simulink model "simpleVehicleModel_Trial2"  (R2017b)
settings: Solver=FixedStepAuto  StartTime=0.0  StopTime=inf  FixedStep=0.01  RelTol=1e-3
values from neighbouring files (symbols this model uses):
  beta_ref = 20*pi/180    (= 0.349065850399)    [initialize_simplemodel_Trial.m]
  g = 9.81    [initialize_simplemodel.m]    (also in initialize_simplemodel_Trial.m; tire_friction_circle.m)
  h = 0.35    [initialize_simplemodel.m]    (also in initialize_simplemodel_Trial.m)
  Izz = 1800    [initialize_simplemodel.m]    (also in initialize_simplemodel_Trial.m = 1400)
  lf = 1.4    [initialize_simplemodel.m]    (also in initialize_simplemodel_Trial.m)
  lr = 1.345    [initialize_simplemodel.m]    (also in initialize_simplemodel_Trial.m)
  m = 1400    [initialize_simplemodel.m]    (also in initialize_simplemodel_Trial.m = 1300; tire_friction_circle.m = 1300)
  r = 0.34    [initialize_simplemodel.m]    (also in initialize_simplemodel_Trial.m)
  tr = 1.684/2    (= 0.842)    [initialize_simplemodel.m]    (also in initialize_simplemodel_Trial.m)
  vx = 10    [initialize_simplemodel_Trial.m]    (also in pp_from_simple_model.m; tire_friction_circle.m = 5)
undefined symbols (not defined in the file or in its folder): DiscIntNeverNeededParam
libraries: simulink x35
(part 1 of 2)
settings Model: Creator=ashwin.ramanujam  LastModifiedBy=gandh

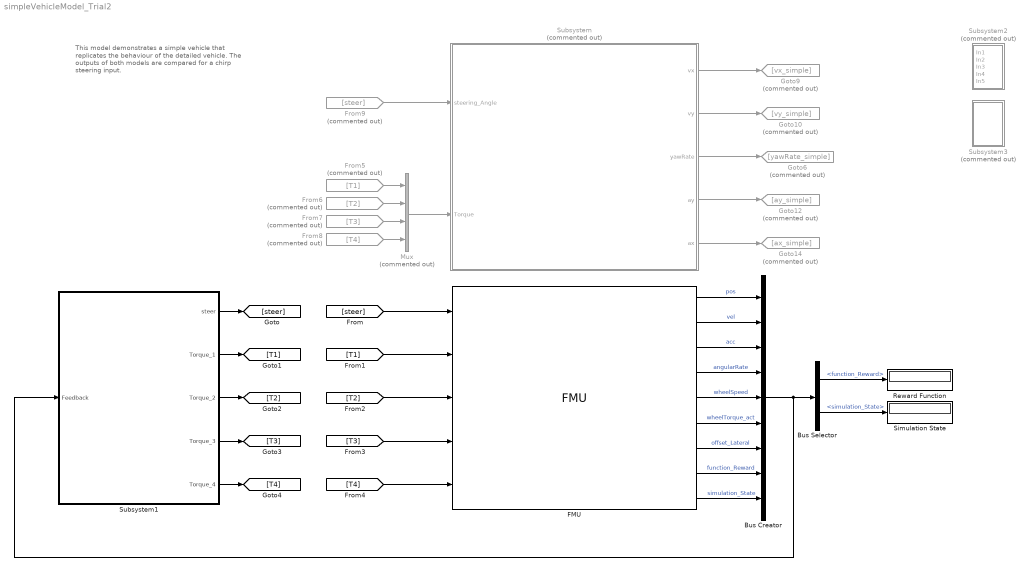
== system simpleVehicleModel_Trial2 ==
  note: This model demonstrates a simple vehicle that replicates the behaviour of the detailed vehicle. The outputs of both models are compared for a chirp steering input.
  Bus Creator : BusCreator  Inputs=9
  Bus Selector : BusSelector  OutputSignals=function_Reward,simulation_State
  FMU : FMU  FMUName=MED2018_VehicleModel.fmu  FMUMode=CoSimulation  FMUSampleTime=-1  mask(MED2018.VehicleModel [Co-Simulation, v2.0]){}
  From5 : From  Commented=on  GotoTag=T1
  From6 : From  Commented=on  GotoTag=T2
  From7 : From  Commented=on  GotoTag=T3
  From8 : From  Commented=on  GotoTag=T4
  From9 : From  Commented=on  GotoTag=steer
  Goto10 : Goto  Commented=on  GotoTag=vy_simple
  Goto12 : Goto  Commented=on  GotoTag=ay_simple
  Goto14 : Goto  Commented=on  GotoTag=ax_simple
  Goto6 : Goto  Commented=on  GotoTag=yawRate_simple
  Goto9 : Goto  Commented=on  GotoTag=vx_simple
  Mux : Mux  Commented=on
  Reward Function : Display
  Simulation State : Display
  Subsystem : Subsystem  Commented=on
  Subsystem1 : Subsystem
  Subsystem2 : Subsystem  Commented=on
  Subsystem3 : Subsystem  Commented=on
  wires:
  Mux/1 -> Subsystem/2(Torque)
  [steer] -> FMU/1
  [T4] -> FMU/5
  [T1] -> FMU/2
  [T2] -> FMU/3
  [T3] -> FMU/4
  From5/1 -> Mux/1
  From6/1 -> Mux/2
  From7/1 -> Mux/3
  From8/1 -> Mux/4
  Subsystem/3(yawRate) -> Goto6/1
  Subsystem/1(vx) -> Goto9/1
  Subsystem/2(vy) -> Goto10/1
  Subsystem/4(ay) -> Goto12/1
  Subsystem/5(ax) -> Goto14/1
  From9/1 -> Subsystem/1(steering_Angle)
  Subsystem1/1(steer) -> [steer]
  Subsystem1/2(Torque_1) -> [T1]
  Subsystem1/3(Torque_2) -> [T2]
  Subsystem1/4(Torque_3) -> [T3]
  Subsystem1/5(Torque_4) -> [T4]
  FMU/1 -> Bus Creator/1  "pos"
  FMU/6 -> Bus Creator/6  "wheelTorque_act"
  FMU/8 -> Bus Creator/8  "function_Reward"
  FMU/3 -> Bus Creator/3  "acc"
  FMU/5 -> Bus Creator/5  "wheelSpeed"
  FMU/7 -> Bus Creator/7  "offset_Lateral"
  FMU/2 -> Bus Creator/2  "vel"
  FMU/4 -> Bus Creator/4  "angularRate"
  FMU/9 -> Bus Creator/9  "simulation_State"
  Bus Creator/1 -> Subsystem1/1(Feedback), Bus Selector/1
  Bus Selector/1 -> Reward Function/1  "<function_Reward>"
  Bus Selector/2 -> Simulation State/1  "<simulation_State>"

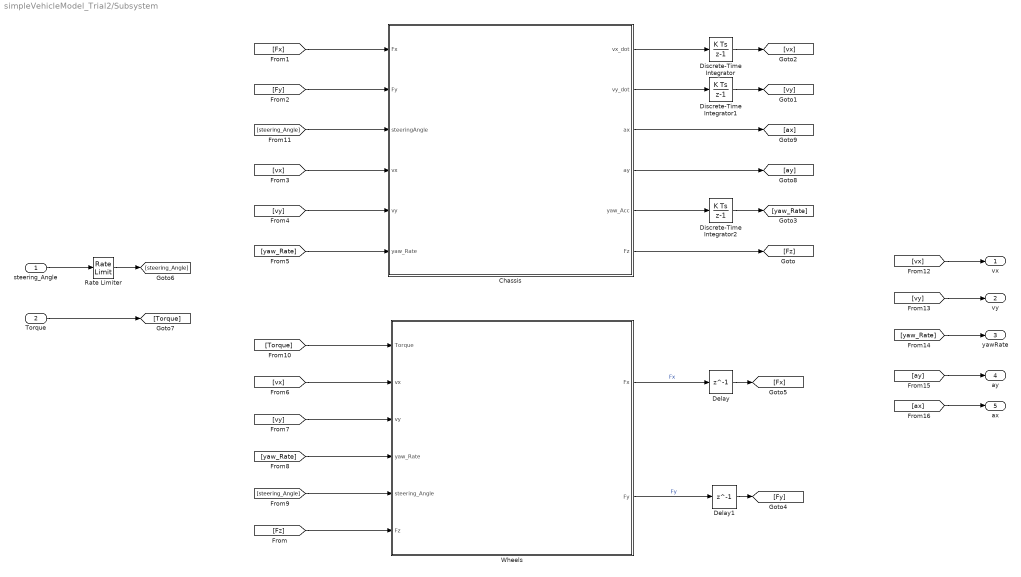
== system simpleVehicleModel_Trial2/Subsystem ==
  steering_Angle : Inport
  Torque : Inport  Port=2
  Chassis : MATLAB Function  TreatAsAtomicUnit=on
  Delay : Delay  DelayLength=1  InitialCondition=[m*g*lr/(lf+lr)/2;m*g*lr/(lf+lr)/2;m*g*lf/(lf+lr)/2;m*g*lf/(lf+lr)/2]
  Delay1 : Delay  DelayLength=1  InitialCondition=[m*g*lr/(lf+lr)/2;m*g*lr/(lf+lr)/2;m*g*lf/(lf+lr)/2;m*g*lf/(lf+lr)/2]
  Discrete-Time Integrator : DiscreteIntegrator  InitialCondition=60*5/18  InitialConditionSetting=State (most efficient)  SampleTime=-1  ICPrevOutput=DiscIntNeverNeededParam  ICPrevScaledInput=DiscIntNeverNeededParam
  Discrete-Time Integrator1 : DiscreteIntegrator  InitialConditionSetting=State (most efficient)  SampleTime=-1  ICPrevOutput=DiscIntNeverNeededParam  ICPrevScaledInput=DiscIntNeverNeededParam
  Discrete-Time Integrator2 : DiscreteIntegrator  InitialConditionSetting=State (most efficient)  SampleTime=-1  ICPrevOutput=DiscIntNeverNeededParam  ICPrevScaledInput=DiscIntNeverNeededParam
  Rate Limiter : RateLimiter  RisingSlewLimit=500*pi/180/12  FallingSlewLimit=-500*pi/180/12  SampleTimeMode=inherited
  Wheels : Subsystem  Priority=0
  vx : Outport
  vy : Outport  Port=2
  yawRate : Outport  Port=3
  ay : Outport  Port=4
  ax : Outport  Port=5
  wires:
  [vx] -> Chassis/4(vx)
  Discrete-Time Integrator2/1 -> [yaw_Rate]
  [Fy] -> Chassis/2(Fy)
  [vy] -> Wheels/3(vy)
  [Torque] -> Wheels/1(Torque)
  [yaw_Rate] -> yawRate/1
  [yaw_Rate] -> Wheels/4(yaw_Rate)
  [vx] -> vx/1
  [vx] -> Wheels/2(vx)
  [Fz] -> Wheels/6(Fz)
  [steering_Angle] -> Chassis/3(steeringAngle)
  [steering_Angle] -> Wheels/5(steering_Angle)
  steering_Angle/1 -> Rate Limiter/1
  Torque/1 -> [Torque]
  [vy] -> vy/1
  Chassis/5(yaw_Acc) -> Discrete-Time Integrator2/1
  Wheels/1(Fx) -> Delay/1  "Fx"
  Wheels/2(Fy) -> Delay1/1  "Fy"
  Chassis/6(Fz) -> [Fz]
  [ay] -> ay/1
  Delay/1 -> [Fx]
  Delay1/1 -> [Fy]
  Chassis/1(vx_dot) -> Discrete-Time Integrator/1
  Chassis/4(ay) -> [ay]
  Chassis/3(ax) -> [ax]
  [ax] -> ax/1
  Chassis/2(vy_dot) -> Discrete-Time Integrator1/1
  [vy] -> Chassis/5(vy)
  [yaw_Rate] -> Chassis/6(yaw_Rate)
  [Fx] -> Chassis/1(Fx)
  Discrete-Time Integrator1/1 -> [vy]
  Discrete-Time Integrator/1 -> [vx]
  Rate Limiter/1 -> [steering_Angle]

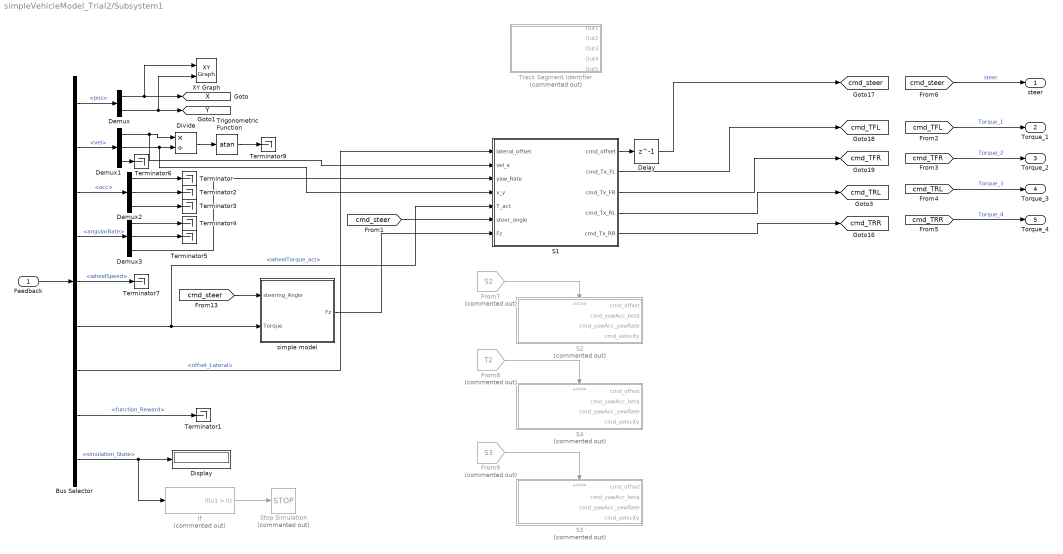
== system simpleVehicleModel_Trial2/Subsystem1 ==
  Feedback : Inport
  Bus Selector : BusSelector  OutputSignals=pos,vel,acc,angularRate,wheelSpeed,wheelTorque_act,offset_Lateral,function_Reward,simulation_State
  Delay : Delay  DelayLength=1
  Demux : Demux  Outputs=2
  Demux1 : Demux  Outputs=3
  Demux2 : Demux  Outputs=3
  Demux3 : Demux  Outputs=3
  Display : Display
  Divide : Product  Inputs=*/
  From7 : From  Commented=on  GotoTag=S2  TagVisibility=global
  From8 : From  Commented=on  GotoTag=T2  TagVisibility=global
  From9 : From  Commented=on  GotoTag=S3  TagVisibility=global
  If : If  Commented=on  ShowElse=off
  S1 : Subsystem  TreatAsAtomicUnit=on
  S2 : Subsystem  Commented=on  TreatAsAtomicUnit=on
  S3 : Subsystem  Commented=on  TreatAsAtomicUnit=on
  S4 : Subsystem  Commented=on  TreatAsAtomicUnit=on
  Stop Simulation : Stop  Commented=on
  Terminator{,1..7,9} (9 alike) : Terminator
  Track Segment Identifier : Subsystem  Commented=on
  Trigonometric Function : Trigonometry  Operator=atan
  XY Graph : simulink/Sinks/XY Graph  xmin=-5  xmax=110  ymin=-10  ymax=180  st=-1
  simple model : Subsystem
  steer : Outport
  Torque_1 : Outport  Port=2
  Torque_2 : Outport  Port=3
  Torque_3 : Outport  Port=4
  Torque_4 : Outport  Port=5
  tag scope: X=global, Y=global, cmd_TFL=global, cmd_TFR=global, cmd_TRL=global, cmd_TRR=global, cmd_steer=global
  wires:
  [cmd_TFL] -> Torque_1/1  "Torque_1"
  [cmd_TRL] -> Torque_3/1  "Torque_3"
  [cmd_TFR] -> Torque_2/1  "Torque_2"
  [cmd_TRR] -> Torque_4/1  "Torque_4"
  [cmd_steer] -> steer/1  "steer"
  Feedback/1 -> Bus Selector/1
  Bus Selector/1 -> Demux/1  "<pos>"
  Demux/2 -> XY Graph/2, [Y]
  Demux/1 -> XY Graph/1, [X]
  Demux1/1 -> S1/2(vel_x), Divide/1
  Bus Selector/2 -> Demux1/1  "<vel>"
  Demux2/3 -> Terminator3/1
  Bus Selector/3 -> Demux2/1  "<acc>"
  Demux2/2 -> Terminator2/1
  Demux2/1 -> Terminator/1
  Demux3/1 -> Terminator4/1
  Demux3/2 -> Terminator5/1
  Bus Selector/4 -> Demux3/1  "<angularRate>"
  Demux3/3 -> S1/3(yaw_Rate)
  Bus Selector/5 -> Terminator7/1  "<wheelSpeed>"
  Bus Selector/8 -> Terminator1/1  "<function_Reward>"
  Bus Selector/9 -> If/1, Display/1  "<simulation_State>"
  Demux1/2 -> S1/4(v_y), Divide/2
  Divide/1 -> Trigonometric Function/1
  Trigonometric Function/1 -> Terminator9/1
  If/1 -> Stop Simulation/1
  From7/1 -> S2/Action
  From8/1 -> S4/Action
  From9/1 -> S3/Action
  Demux1/3 -> Terminator6/1
  Bus Selector/6 -> S1/5(T_act), simple model/2(Torque)  "<wheelTorque_act>"
  [cmd_steer] -> simple model/1(steering_Angle)
  [cmd_steer] -> S1/6(steer_angle)
  simple model/1(Fz) -> S1/7(Fz)
  Bus Selector/7 -> S1/1(lateral_offset)  "<offset_Lateral>"
  S1/2(cmd_Tx_FL) -> [cmd_TFL]
  S1/3(cmd_Tx_FR) -> [cmd_TFR]
  S1/4(cmd_Tx_RL) -> [cmd_TRL]
  S1/5(cmd_Tx_RR) -> [cmd_TRR]
  S1/1(cmd_offset) -> Delay/1
  Delay/1 -> [cmd_steer]

== system simpleVehicleModel_Trial2/Subsystem2 ==
  In1 : Inport
  In2 : Inport  Port=2
  In3 : Inport  Port=3
  In4 : Inport  Port=4
  In5 : Inport  Port=5
  Demux : Demux  Commented=on  Outputs=3
  Demux1 : Demux  Commented=on  Outputs=3
  Demux2 : Demux  Commented=on  Outputs=3
  Demux3 : Demux  Commented=on  Outputs=2
  Goto11 : Goto  Commented=on  GotoTag=ay_FMU
  Goto13 : Goto  Commented=on  GotoTag=ax_FMU
  Goto15 : Goto  Commented=on  GotoTag=offset_Lateral  TagVisibility=global
  Goto5 : Goto  Commented=on  GotoTag=yawRate_FMU
  Goto7 : Goto  Commented=on  GotoTag=vx_FMU
  Goto8 : Goto  Commented=on  GotoTag=vy_FMU
  Terminator{,2..4} (4 alike) : Terminator  Commented=on
  XY Graph : simulink/Sinks/XY Graph  Commented=on  xmin=-5  xmax=110  ymin=-10  ymax=180  st=-1
  wires:
  Demux/3 -> Goto5/1
  Demux1/1 -> Goto7/1
  Demux1/2 -> Goto8/1
  Demux/1 -> Terminator3/1
  Demux/2 -> Terminator4/1
  Demux2/2 -> Goto11/1
  Demux1/3 -> Terminator/1
  Demux2/1 -> Goto13/1
  Demux3/1 -> XY Graph/1
  Demux3/2 -> XY Graph/2
  Demux2/3 -> Terminator2/1
  In5/1 -> Goto15/1
  In2/1 -> Demux1/1
  In4/1 -> Demux/1
  In1/1 -> Demux3/1
  In3/1 -> Demux2/1

== system simpleVehicleModel_Trial2/Subsystem3 ==
  Scope{,1..3,5} (5 alike) : Scope  NumInputPorts=2
  wires:
  [vx_simple] -> Scope/1  "vx_simple"
  [vx_FMU] -> Scope/2  "vx_FMU"
  [vy_FMU] -> Scope1/2  "vy_FMU"
  [vy_simple] -> Scope1/1  "vy_simple"
  [ax_FMU] -> Scope5/2  "ax_FMU"
  [yawRate_simple] -> Scope2/1  "yawRate_simple"
  [yawRate_FMU] -> Scope2/2  "yawRate_FMU"
  [ay_simple] -> Scope3/1  "ay_simple"
  [ay_FMU] -> Scope3/2  "ay_FMU"
  [ax_simple] -> Scope5/1  "ax_simple"

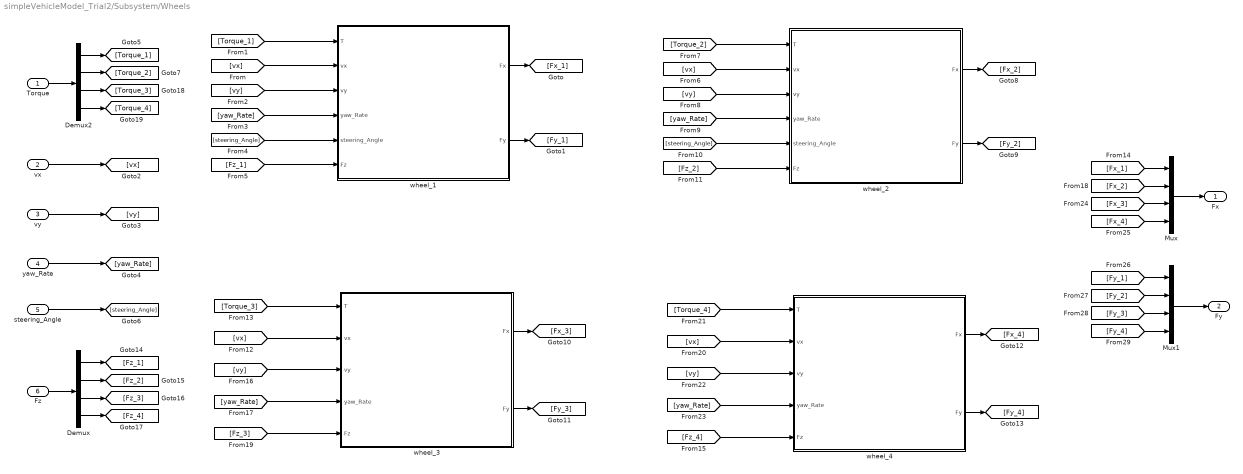
== system simpleVehicleModel_Trial2/Subsystem/Wheels ==
  Torque : Inport
  vx : Inport  Port=2
  vy : Inport  Port=3
  yaw_Rate : Inport  Port=4
  steering_Angle : Inport  Port=5
  Fz : Inport  Port=6
  Demux : Demux
  Demux2 : Demux
  Mux : Mux
  Mux1 : Mux
  wheel_1 : Subsystem
  wheel_2 : Subsystem
  wheel_3 : Subsystem
  wheel_4 : Subsystem
  Fx : Outport
  Fy : Outport  Port=2
  wires:
  vx/1 -> [vx]
  vy/1 -> [vy]
  yaw_Rate/1 -> [yaw_Rate]
  [vx] -> wheel_1/2(vx)
  wheel_1/1(Fx) -> [Fx_1]
  wheel_1/2(Fy) -> [Fy_1]
  [steering_Angle] -> wheel_1/5(steering_Angle)
  [yaw_Rate] -> wheel_1/4(yaw_Rate)
  [vy] -> wheel_1/3(vy)
  [Torque_1] -> wheel_1/1(T)
  steering_Angle/1 -> [steering_Angle]
  wheel_2/1(Fx) -> [Fx_2]
  wheel_2/2(Fy) -> [Fy_2]
  [yaw_Rate] -> wheel_2/4(yaw_Rate)
  [vy] -> wheel_2/3(vy)
  [steering_Angle] -> wheel_2/5(steering_Angle)
  [vx] -> wheel_2/2(vx)
  wheel_3/1(Fx) -> [Fx_3]
  [yaw_Rate] -> wheel_3/4(yaw_Rate)
  [vy] -> wheel_4/3(vy)
  [yaw_Rate] -> wheel_4/4(yaw_Rate)
  [vx] -> wheel_4/2(vx)
  wheel_4/2(Fy) -> [Fy_4]
  wheel_3/2(Fy) -> [Fy_3]
  wheel_4/1(Fx) -> [Fx_4]
  [vy] -> wheel_3/3(vy)
  [vx] -> wheel_3/2(vx)
  [Fx_1] -> Mux/1
  [Fx_2] -> Mux/2
  [Fx_3] -> Mux/3
  [Fx_4] -> Mux/4
  [Fy_3] -> Mux1/3
  [Fy_4] -> Mux1/4
  [Fy_2] -> Mux1/2
  [Fy_1] -> Mux1/1
  Demux/1 -> [Fz_1]
  Demux/2 -> [Fz_2]
  Demux/3 -> [Fz_3]
  Demux/4 -> [Fz_4]
  [Fz_1] -> wheel_1/6(Fz)
  [Fz_3] -> wheel_3/5(Fz)
  [Fz_4] -> wheel_4/5(Fz)
  [Fz_2] -> wheel_2/6(Fz)
  Fz/1 -> Demux/1
  [Torque_3] -> wheel_3/1(T)
  [Torque_2] -> wheel_2/1(T)
  [Torque_4] -> wheel_4/1(T)
  Demux2/4 -> [Torque_4]
  Demux2/3 -> [Torque_3]
  Demux2/1 -> [Torque_1]
  Torque/1 -> Demux2/1
  Demux2/2 -> [Torque_2]
  Mux1/1 -> Fy/1
  Mux/1 -> Fx/1

== system simpleVehicleModel_Trial2/Subsystem1/S1 ==
  lateral_offset : Inport
  vel_x : Inport  Port=2
  yaw_Rate : Inport  Port=3
  v_y : Inport  Port=4
  T_act : Inport  Port=5
  steer_angle : Inport  Port=6
  Fz : Inport  Port=7
  Constant4 : Constant  Value=0
  Discrete PID Controller : simulink/Continuous/PID Controller  Controller=PID  TimeDomain=Discrete-time  SampleTime=-1  IntegratorMethod=Forward Euler  FilterMethod=Forward Euler  Form=Parallel  UseFilter=off  ControllerParametersSource=internal  P=1  I=0  D=1  N=100  InitialConditionSource=internal  InitialConditionForIntegrator=0  InitialConditionForFilter=0  ExternalReset=none  LimitOutput=off  UpperSaturationLimit=inf  LowerSaturationLimit=-inf  LinearizeAsGain=off  AntiWindupMode=none  Kb=1  TrackingMode=off  Kt=1  PParamMin=[]  PParamMax=[]  IParamMin=[]  IParamMax=[]  DParamMin=[]  DParamMax=[]  NParamMin=[]  NParamMax=[]  KbParamMin=[]  KbParamMax=[]  KtParamMin=[]  KtParamMax=[]  POutMin=[]  POutMax=[]  IOutMin=[]  IOutMax=[]  DOutMin=[]  DOutMax=[]  NOutMin=[]  NOutMax=[]  KbOutMin=[]  KbOutMax=[]  KtOutMin=[]  KtOutMax=[]  IntegratorOutMin=[]  IntegratorOutMax=[]  FilterOutMin=[]  FilterOutMax=[]  SumOutMin=[]  SumOutMax=[]  SumI1OutMin=[]  SumI1OutMax=[]  SumI2OutMin=[]  SumI2OutMax=[]  SumI3OutMin=[]  SumI3OutMax=[]  SumDOutMin=[]  SumDOutMax=[]  SaturationOutMin=[]  SaturationOutMax=[]  IntegratorContinuousStateAttributes=''  IntegratorStateMustResolveToSignalObject=off  IntegratorRTWStateStorageClass=Auto  FilterContinuousStateAttributes=''  FilterStateMustResolveToSignalObject=off  FilterRTWStateStorageClass=Auto  DifferentiatorICPrevScaledInput=0  DifferentiatorOutMin=[]  DifferentiatorOutMax=[]  InitialConditionSetting=State (most efficient)  FilterDiffOutCoefMin=[]  FilterDiffOutCoefMax=[]  SumDenOutMin=[]  SumDenOutMax=[]  SumNumOutMin=[]  SumNumOutMax=[]  ReciprocalOutMin=[]  ReciprocalOutMax=[]  DivideOutMin=[]  DivideOutMax=[]  TunerSelectOption=Transfer Function Based (PID Tuner App)
  Discrete PID Controller5 : simulink/Continuous/PID Controller  Controller=PID  TimeDomain=Discrete-time  SampleTime=-1  IntegratorMethod=Forward Euler  FilterMethod=Forward Euler  Form=Parallel  UseFilter=off  ControllerParametersSource=internal  P=200  I=0  D=1  N=100  InitialConditionSource=internal  InitialConditionForIntegrator=0  InitialConditionForFilter=0  ExternalReset=none  LimitOutput=off  UpperSaturationLimit=inf  LowerSaturationLimit=-inf  LinearizeAsGain=off  AntiWindupMode=none  Kb=1  TrackingMode=off  Kt=1  PParamMin=[]  PParamMax=[]  IParamMin=[]  IParamMax=[]  DParamMin=[]  DParamMax=[]  NParamMin=[]  NParamMax=[]  KbParamMin=[]  KbParamMax=[]  KtParamMin=[]  KtParamMax=[]  POutMin=[]  POutMax=[]  IOutMin=[]  IOutMax=[]  DOutMin=[]  DOutMax=[]  NOutMin=[]  NOutMax=[]  KbOutMin=[]  KbOutMax=[]  KtOutMin=[]  KtOutMax=[]  IntegratorOutMin=[]  IntegratorOutMax=[]  FilterOutMin=[]  FilterOutMax=[]  SumOutMin=[]  SumOutMax=[]  SumI1OutMin=[]  SumI1OutMax=[]  SumI2OutMin=[]  SumI2OutMax=[]  SumI3OutMin=[]  SumI3OutMax=[]  SumDOutMin=[]  SumDOutMax=[]  SaturationOutMin=[]  SaturationOutMax=[]  IntegratorContinuousStateAttributes=''  IntegratorStateMustResolveToSignalObject=off  IntegratorRTWStateStorageClass=Auto  FilterContinuousStateAttributes=''  FilterStateMustResolveToSignalObject=off  FilterRTWStateStorageClass=Auto  DifferentiatorICPrevScaledInput=0  DifferentiatorOutMin=[]  DifferentiatorOutMax=[]  InitialConditionSetting=State (most efficient)  FilterDiffOutCoefMin=[]  FilterDiffOutCoefMax=[]  SumDenOutMin=[]  SumDenOutMax=[]  SumNumOutMin=[]  SumNumOutMax=[]  ReciprocalOutMin=[]  ReciprocalOutMax=[]  DivideOutMin=[]  DivideOutMax=[]  TunerSelectOption=Transfer Function Based (PID Tuner App)
  Gain : Gain  Gain=r
  Subtract3 : Sum  Inputs=+-
  Subtract5 : Sum  Inputs=+-
  Wheel Traction control : Subsystem
  Wheels : Subsystem  Priority=0
  ref_velocity : Constant  Value=vx
  cmd_offset : Outport
  cmd_Tx_FL : Outport  Port=2
  cmd_Tx_FR : Outport  Port=3
  cmd_Tx_RL : Outport  Port=4
  cmd_Tx_RR : Outport  Port=5
  wires:
  Subtract5/1 -> Discrete PID Controller5/1  "velocity_error"
  ref_velocity/1 -> Subtract5/1
  vel_x/1 -> Wheels/2(vx), Subtract5/2
  Constant4/1 -> Subtract3/1  "ref_offset"
  Subtract3/1 -> Discrete PID Controller/1  "offset_error"
  lateral_offset/1 -> Subtract3/2
  Discrete PID Controller/1 -> cmd_offset/1  "cmd_offset"
  T_act/1 -> Wheels/1(Torque)
  v_y/1 -> Wheels/3(vy)
  yaw_Rate/1 -> Wheels/4(yaw_Rate)
  steer_angle/1 -> Wheels/5(steering_Angle)
  Fz/1 -> Wheels/6(Fz)
  Wheels/1(Fxmargin) -> Gain/1
  Discrete PID Controller5/1 -> Wheel Traction control/1(cmd_Tx)  "cmd_Tx"
  Gain/1 -> Wheel Traction control/2(Fmargin)
  Wheel Traction control/1(cmd_Tx_FL) -> cmd_Tx_FL/1
  Wheel Traction control/2(cmd_Tx_FR) -> cmd_Tx_FR/1
  Wheel Traction control/3(cmd_Tx_RL) -> cmd_Tx_RL/1
  Wheel Traction control/4(cmd_Tx_RR) -> cmd_Tx_RR/1

== system simpleVehicleModel_Trial2/Subsystem1/S2 ==
  Action Port : ActionPort
  Constant4 : Constant  Value=0
  Discrete Derivative : simulink/Discrete/Discrete Derivative  gainval=1.0  ICPrevScaledInput=0.0  OutMin=[]  OutMax=[]  OutDataType=fixdt(1, 16)  OutScaling=2^-10  DoSatur=off
  Discrete PID Controller : simulink/Continuous/PID Controller  Controller=PID  TimeDomain=Discrete-time  SampleTime=-1  IntegratorMethod=Forward Euler  FilterMethod=Forward Euler  Form=Parallel  UseFilter=on  ControllerParametersSource=internal  P=1  I=0  D=0.1  N=100  InitialConditionSource=internal  InitialConditionForIntegrator=0  InitialConditionForFilter=0  ExternalReset=none  LimitOutput=off  UpperSaturationLimit=inf  LowerSaturationLimit=-inf  LinearizeAsGain=off  AntiWindupMode=none  Kb=1  TrackingMode=off  Kt=1  PParamMin=[]  PParamMax=[]  IParamMin=[]  IParamMax=[]  DParamMin=[]  DParamMax=[]  NParamMin=[]  NParamMax=[]  KbParamMin=[]  KbParamMax=[]  KtParamMin=[]  KtParamMax=[]  POutMin=[]  POutMax=[]  IOutMin=[]  IOutMax=[]  DOutMin=[]  DOutMax=[]  NOutMin=[]  NOutMax=[]  KbOutMin=[]  KbOutMax=[]  KtOutMin=[]  KtOutMax=[]  IntegratorOutMin=[]  IntegratorOutMax=[]  FilterOutMin=[]  FilterOutMax=[]  SumOutMin=[]  SumOutMax=[]  SumI1OutMin=[]  SumI1OutMax=[]  SumI2OutMin=[]  SumI2OutMax=[]  SumI3OutMin=[]  SumI3OutMax=[]  SumDOutMin=[]  SumDOutMax=[]  SaturationOutMin=[]  SaturationOutMax=[]  IntegratorContinuousStateAttributes=''  IntegratorStateMustResolveToSignalObject=off  IntegratorRTWStateStorageClass=Auto  FilterContinuousStateAttributes=''  FilterStateMustResolveToSignalObject=off  FilterRTWStateStorageClass=Auto  DifferentiatorICPrevScaledInput=0  DifferentiatorOutMin=[]  DifferentiatorOutMax=[]  InitialConditionSetting=State (most efficient)  FilterDiffOutCoefMin=[]  FilterDiffOutCoefMax=[]  SumDenOutMin=[]  SumDenOutMax=[]  SumNumOutMin=[]  SumNumOutMax=[]  ReciprocalOutMin=[]  ReciprocalOutMax=[]  DivideOutMin=[]  DivideOutMax=[]  TunerSelectOption=Transfer Function Based (PID Tuner App)
  Discrete PID Controller{1..5} (5 alike) : simulink/Continuous/PID Controller  Controller=PID  TimeDomain=Discrete-time  SampleTime=-1  IntegratorMethod=Forward Euler  FilterMethod=Forward Euler  Form=Parallel  UseFilter=on  ControllerParametersSource=internal  P=1  I=1  D=0  N=100  InitialConditionSource=internal  InitialConditionForIntegrator=0  InitialConditionForFilter=0  ExternalReset=none  LimitOutput=off  UpperSaturationLimit=inf  LowerSaturationLimit=-inf  LinearizeAsGain=off  AntiWindupMode=none  Kb=1  TrackingMode=off  Kt=1  PParamMin=[]  PParamMax=[]  IParamMin=[]  IParamMax=[]  DParamMin=[]  DParamMax=[]  NParamMin=[]  NParamMax=[]  KbParamMin=[]  KbParamMax=[]  KtParamMin=[]  KtParamMax=[]  POutMin=[]  POutMax=[]  IOutMin=[]  IOutMax=[]  DOutMin=[]  DOutMax=[]  NOutMin=[]  NOutMax=[]  KbOutMin=[]  KbOutMax=[]  KtOutMin=[]  KtOutMax=[]  IntegratorOutMin=[]  IntegratorOutMax=[]  FilterOutMin=[]  FilterOutMax=[]  SumOutMin=[]  SumOutMax=[]  SumI1OutMin=[]  SumI1OutMax=[]  SumI2OutMin=[]  SumI2OutMax=[]  SumI3OutMin=[]  SumI3OutMax=[]  SumDOutMin=[]  SumDOutMax=[]  SaturationOutMin=[]  SaturationOutMax=[]  IntegratorContinuousStateAttributes=''  IntegratorStateMustResolveToSignalObject=off  IntegratorRTWStateStorageClass=Auto  FilterContinuousStateAttributes=''  FilterStateMustResolveToSignalObject=off  FilterRTWStateStorageClass=Auto  DifferentiatorICPrevScaledInput=0  DifferentiatorOutMin=[]  DifferentiatorOutMax=[]  InitialConditionSetting=State (most efficient)  FilterDiffOutCoefMin=[]  FilterDiffOutCoefMax=[]  SumDenOutMin=[]  SumDenOutMax=[]  SumNumOutMin=[]  SumNumOutMax=[]  ReciprocalOutMin=[]  ReciprocalOutMax=[]  DivideOutMin=[]  DivideOutMax=[]  TunerSelectOption=Transfer Function Based (PID Tuner App)
  Subtract{,1..5} (6 alike) : Sum  Inputs=+-
  beta_ref : Constant  Value=beta_ref
  ref_velocity : Constant  Value=vx
  yawrate_ref : Constant  Value=vx/r
  cmd_offset : Outport
  cmd_yawAcc_beta : Outport  Port=2
  cmd_yawAcc_yawRate : Outport  Port=3
  cmd_velocity : Outport  Port=4
  wires:
  Discrete PID Controller5/1 -> cmd_velocity/1  "cmd_velocity"
  Subtract5/1 -> Discrete PID Controller5/1
  ref_velocity/1 -> Subtract5/1
  [vel_X] -> Subtract5/2
  Discrete Derivative/1 -> Subtract2/2, Subtract4/2
  Constant4/1 -> Subtract3/1  "ref_offset"
  Discrete PID Controller3/1 -> cmd_yawAcc_beta/1  "cmd_yawAcc_beta"
  Subtract/1 -> Discrete PID Controller1/1  "beta_error"
  Subtract4/1 -> Discrete PID Controller4/1
  beta_ref/1 -> Subtract/1
  Discrete PID Controller2/1 -> Subtract4/1  "yawAcc_ref2"
  Subtract3/1 -> Discrete PID Controller/1  "offset_error"
  [yawRate] -> Subtract1/2, Discrete Derivative/1
  Discrete PID Controller1/1 -> Subtract2/1  "yawAcc_ref1"
  yawrate_ref/1 -> Subtract1/1
  Subtract2/1 -> Discrete PID Controller3/1
  [offset_Lateral] -> Subtract3/2
  Discrete PID Controller/1 -> cmd_offset/1  "cmd_offset"
  [beta] -> Subtract/2
  Subtract1/1 -> Discrete PID Controller2/1  "yawRate_error"
  Discrete PID Controller4/1 -> cmd_yawAcc_yawRate/1  "cmd_yawAcc_yawRate"

== system simpleVehicleModel_Trial2/Subsystem1/S3 ==
  Action Port : ActionPort
  Constant4 : Constant  Value=0
  Discrete Derivative : simulink/Discrete/Discrete Derivative  gainval=1.0  ICPrevScaledInput=0.0  OutMin=[]  OutMax=[]  OutDataType=fixdt(1, 16)  OutScaling=2^-10  DoSatur=off
  Discrete PID Controller : simulink/Continuous/PID Controller  Controller=PID  TimeDomain=Discrete-time  SampleTime=-1  IntegratorMethod=Forward Euler  FilterMethod=Forward Euler  Form=Parallel  UseFilter=on  ControllerParametersSource=internal  P=1  I=0  D=0.1  N=100  InitialConditionSource=internal  InitialConditionForIntegrator=0  InitialConditionForFilter=0  ExternalReset=none  LimitOutput=off  UpperSaturationLimit=inf  LowerSaturationLimit=-inf  LinearizeAsGain=off  AntiWindupMode=none  Kb=1  TrackingMode=off  Kt=1  PParamMin=[]  PParamMax=[]  IParamMin=[]  IParamMax=[]  DParamMin=[]  DParamMax=[]  NParamMin=[]  NParamMax=[]  KbParamMin=[]  KbParamMax=[]  KtParamMin=[]  KtParamMax=[]  POutMin=[]  POutMax=[]  IOutMin=[]  IOutMax=[]  DOutMin=[]  DOutMax=[]  NOutMin=[]  NOutMax=[]  KbOutMin=[]  KbOutMax=[]  KtOutMin=[]  KtOutMax=[]  IntegratorOutMin=[]  IntegratorOutMax=[]  FilterOutMin=[]  FilterOutMax=[]  SumOutMin=[]  SumOutMax=[]  SumI1OutMin=[]  SumI1OutMax=[]  SumI2OutMin=[]  SumI2OutMax=[]  SumI3OutMin=[]  SumI3OutMax=[]  SumDOutMin=[]  SumDOutMax=[]  SaturationOutMin=[]  SaturationOutMax=[]  IntegratorContinuousStateAttributes=''  IntegratorStateMustResolveToSignalObject=off  IntegratorRTWStateStorageClass=Auto  FilterContinuousStateAttributes=''  FilterStateMustResolveToSignalObject=off  FilterRTWStateStorageClass=Auto  DifferentiatorICPrevScaledInput=0  DifferentiatorOutMin=[]  DifferentiatorOutMax=[]  InitialConditionSetting=State (most efficient)  FilterDiffOutCoefMin=[]  FilterDiffOutCoefMax=[]  SumDenOutMin=[]  SumDenOutMax=[]  SumNumOutMin=[]  SumNumOutMax=[]  ReciprocalOutMin=[]  ReciprocalOutMax=[]  DivideOutMin=[]  DivideOutMax=[]  TunerSelectOption=Transfer Function Based (PID Tuner App)
  Discrete PID Controller{1..5} (5 alike) : simulink/Continuous/PID Controller  Controller=PID  TimeDomain=Discrete-time  SampleTime=-1  IntegratorMethod=Forward Euler  FilterMethod=Forward Euler  Form=Parallel  UseFilter=on  ControllerParametersSource=internal  P=1  I=1  D=0  N=100  InitialConditionSource=internal  InitialConditionForIntegrator=0  InitialConditionForFilter=0  ExternalReset=none  LimitOutput=off  UpperSaturationLimit=inf  LowerSaturationLimit=-inf  LinearizeAsGain=off  AntiWindupMode=none  Kb=1  TrackingMode=off  Kt=1  PParamMin=[]  PParamMax=[]  IParamMin=[]  IParamMax=[]  DParamMin=[]  DParamMax=[]  NParamMin=[]  NParamMax=[]  KbParamMin=[]  KbParamMax=[]  KtParamMin=[]  KtParamMax=[]  POutMin=[]  POutMax=[]  IOutMin=[]  IOutMax=[]  DOutMin=[]  DOutMax=[]  NOutMin=[]  NOutMax=[]  KbOutMin=[]  KbOutMax=[]  KtOutMin=[]  KtOutMax=[]  IntegratorOutMin=[]  IntegratorOutMax=[]  FilterOutMin=[]  FilterOutMax=[]  SumOutMin=[]  SumOutMax=[]  SumI1OutMin=[]  SumI1OutMax=[]  SumI2OutMin=[]  SumI2OutMax=[]  SumI3OutMin=[]  SumI3OutMax=[]  SumDOutMin=[]  SumDOutMax=[]  SaturationOutMin=[]  SaturationOutMax=[]  IntegratorContinuousStateAttributes=''  IntegratorStateMustResolveToSignalObject=off  IntegratorRTWStateStorageClass=Auto  FilterContinuousStateAttributes=''  FilterStateMustResolveToSignalObject=off  FilterRTWStateStorageClass=Auto  DifferentiatorICPrevScaledInput=0  DifferentiatorOutMin=[]  DifferentiatorOutMax=[]  InitialConditionSetting=State (most efficient)  FilterDiffOutCoefMin=[]  FilterDiffOutCoefMax=[]  SumDenOutMin=[]  SumDenOutMax=[]  SumNumOutMin=[]  SumNumOutMax=[]  ReciprocalOutMin=[]  ReciprocalOutMax=[]  DivideOutMin=[]  DivideOutMax=[]  TunerSelectOption=Transfer Function Based (PID Tuner App)
  Subtract{,1..5} (6 alike) : Sum  Inputs=+-
  beta_ref : Constant  Value=beta_ref
  ref_velocity : Constant  Value=vx
  yawrate_ref : Constant  Value=vx/r
  cmd_offset : Outport
  cmd_yawAcc_beta : Outport  Port=2
  cmd_yawAcc_yawRate : Outport  Port=3
  cmd_velocity : Outport  Port=4
  wires:
  Discrete PID Controller5/1 -> cmd_velocity/1  "cmd_velocity"
  Subtract5/1 -> Discrete PID Controller5/1
  ref_velocity/1 -> Subtract5/1
  [vel_X] -> Subtract5/2
  Discrete Derivative/1 -> Subtract2/2, Subtract4/2
  Constant4/1 -> Subtract3/1  "ref_offset"
  Discrete PID Controller3/1 -> cmd_yawAcc_beta/1  "cmd_yawAcc_beta"
  Subtract/1 -> Discrete PID Controller1/1  "beta_error"
  Subtract4/1 -> Discrete PID Controller4/1
  beta_ref/1 -> Subtract/1
  Discrete PID Controller2/1 -> Subtract4/1  "yawAcc_ref2"
  Subtract3/1 -> Discrete PID Controller/1  "offset_error"
  [yawRate] -> Subtract1/2, Discrete Derivative/1
  Discrete PID Controller1/1 -> Subtract2/1  "yawAcc_ref1"
  yawrate_ref/1 -> Subtract1/1
  Subtract2/1 -> Discrete PID Controller3/1
  [offset_Lateral] -> Subtract3/2
  Discrete PID Controller/1 -> cmd_offset/1  "cmd_offset"
  [beta] -> Subtract/2
  Subtract1/1 -> Discrete PID Controller2/1  "yawRate_error"
  Discrete PID Controller4/1 -> cmd_yawAcc_yawRate/1  "cmd_yawAcc_yawRate"

== system simpleVehicleModel_Trial2/Subsystem1/S4 ==
  Action Port : ActionPort
  Constant4 : Constant  Value=0
  Discrete Derivative : simulink/Discrete/Discrete Derivative  gainval=1.0  ICPrevScaledInput=0.0  OutMin=[]  OutMax=[]  OutDataType=fixdt(1, 16)  OutScaling=2^-10  DoSatur=off
  Discrete PID Controller : simulink/Continuous/PID Controller  Controller=PID  TimeDomain=Discrete-time  SampleTime=-1  IntegratorMethod=Forward Euler  FilterMethod=Forward Euler  Form=Parallel  UseFilter=on  ControllerParametersSource=internal  P=1  I=0  D=0.1  N=100  InitialConditionSource=internal  InitialConditionForIntegrator=0  InitialConditionForFilter=0  ExternalReset=none  LimitOutput=off  UpperSaturationLimit=inf  LowerSaturationLimit=-inf  LinearizeAsGain=off  AntiWindupMode=none  Kb=1  TrackingMode=off  Kt=1  PParamMin=[]  PParamMax=[]  IParamMin=[]  IParamMax=[]  DParamMin=[]  DParamMax=[]  NParamMin=[]  NParamMax=[]  KbParamMin=[]  KbParamMax=[]  KtParamMin=[]  KtParamMax=[]  POutMin=[]  POutMax=[]  IOutMin=[]  IOutMax=[]  DOutMin=[]  DOutMax=[]  NOutMin=[]  NOutMax=[]  KbOutMin=[]  KbOutMax=[]  KtOutMin=[]  KtOutMax=[]  IntegratorOutMin=[]  IntegratorOutMax=[]  FilterOutMin=[]  FilterOutMax=[]  SumOutMin=[]  SumOutMax=[]  SumI1OutMin=[]  SumI1OutMax=[]  SumI2OutMin=[]  SumI2OutMax=[]  SumI3OutMin=[]  SumI3OutMax=[]  SumDOutMin=[]  SumDOutMax=[]  SaturationOutMin=[]  SaturationOutMax=[]  IntegratorContinuousStateAttributes=''  IntegratorStateMustResolveToSignalObject=off  IntegratorRTWStateStorageClass=Auto  FilterContinuousStateAttributes=''  FilterStateMustResolveToSignalObject=off  FilterRTWStateStorageClass=Auto  DifferentiatorICPrevScaledInput=0  DifferentiatorOutMin=[]  DifferentiatorOutMax=[]  InitialConditionSetting=State (most efficient)  FilterDiffOutCoefMin=[]  FilterDiffOutCoefMax=[]  SumDenOutMin=[]  SumDenOutMax=[]  SumNumOutMin=[]  SumNumOutMax=[]  ReciprocalOutMin=[]  ReciprocalOutMax=[]  DivideOutMin=[]  DivideOutMax=[]  TunerSelectOption=Transfer Function Based (PID Tuner App)
  Discrete PID Controller{1..5} (5 alike) : simulink/Continuous/PID Controller  Controller=PID  TimeDomain=Discrete-time  SampleTime=-1  IntegratorMethod=Forward Euler  FilterMethod=Forward Euler  Form=Parallel  UseFilter=on  ControllerParametersSource=internal  P=1  I=1  D=0  N=100  InitialConditionSource=internal  InitialConditionForIntegrator=0  InitialConditionForFilter=0  ExternalReset=none  LimitOutput=off  UpperSaturationLimit=inf  LowerSaturationLimit=-inf  LinearizeAsGain=off  AntiWindupMode=none  Kb=1  TrackingMode=off  Kt=1  PParamMin=[]  PParamMax=[]  IParamMin=[]  IParamMax=[]  DParamMin=[]  DParamMax=[]  NParamMin=[]  NParamMax=[]  KbParamMin=[]  KbParamMax=[]  KtParamMin=[]  KtParamMax=[]  POutMin=[]  POutMax=[]  IOutMin=[]  IOutMax=[]  DOutMin=[]  DOutMax=[]  NOutMin=[]  NOutMax=[]  KbOutMin=[]  KbOutMax=[]  KtOutMin=[]  KtOutMax=[]  IntegratorOutMin=[]  IntegratorOutMax=[]  FilterOutMin=[]  FilterOutMax=[]  SumOutMin=[]  SumOutMax=[]  SumI1OutMin=[]  SumI1OutMax=[]  SumI2OutMin=[]  SumI2OutMax=[]  SumI3OutMin=[]  SumI3OutMax=[]  SumDOutMin=[]  SumDOutMax=[]  SaturationOutMin=[]  SaturationOutMax=[]  IntegratorContinuousStateAttributes=''  IntegratorStateMustResolveToSignalObject=off  IntegratorRTWStateStorageClass=Auto  FilterContinuousStateAttributes=''  FilterStateMustResolveToSignalObject=off  FilterRTWStateStorageClass=Auto  DifferentiatorICPrevScaledInput=0  DifferentiatorOutMin=[]  DifferentiatorOutMax=[]  InitialConditionSetting=State (most efficient)  FilterDiffOutCoefMin=[]  FilterDiffOutCoefMax=[]  SumDenOutMin=[]  SumDenOutMax=[]  SumNumOutMin=[]  SumNumOutMax=[]  ReciprocalOutMin=[]  ReciprocalOutMax=[]  DivideOutMin=[]  DivideOutMax=[]  TunerSelectOption=Transfer Function Based (PID Tuner App)
  Subtract{,1..5} (6 alike) : Sum  Inputs=+-
  beta_ref : Constant  Value=beta_ref
  ref_velocity : Constant  Value=vx
  yawrate_ref : Constant  Value=vx/r
  cmd_offset : Outport
  cmd_yawAcc_beta : Outport  Port=2
  cmd_yawAcc_yawRate : Outport  Port=3
  cmd_velocity : Outport  Port=4
  wires:
  Discrete PID Controller5/1 -> cmd_velocity/1  "cmd_velocity"
  Subtract5/1 -> Discrete PID Controller5/1
  ref_velocity/1 -> Subtract5/1
  [vel_X] -> Subtract5/2
  Discrete Derivative/1 -> Subtract2/2, Subtract4/2
  Constant4/1 -> Subtract3/1  "ref_offset"
  Discrete PID Controller3/1 -> cmd_yawAcc_beta/1  "cmd_yawAcc_beta"
  Subtract/1 -> Discrete PID Controller1/1  "beta_error"
  Subtract4/1 -> Discrete PID Controller4/1
  beta_ref/1 -> Subtract/1
  Discrete PID Controller2/1 -> Subtract4/1  "yawAcc_ref2"
  Subtract3/1 -> Discrete PID Controller/1  "offset_error"
  [yawRate] -> Subtract1/2, Discrete Derivative/1
  Discrete PID Controller1/1 -> Subtract2/1  "yawAcc_ref1"
  yawrate_ref/1 -> Subtract1/1
  Subtract2/1 -> Discrete PID Controller3/1
  [offset_Lateral] -> Subtract3/2
  Discrete PID Controller/1 -> cmd_offset/1  "cmd_offset"
  [beta] -> Subtract/2
  Subtract1/1 -> Discrete PID Controller2/1  "yawRate_error"
  Discrete PID Controller4/1 -> cmd_yawAcc_yawRate/1  "cmd_yawAcc_yawRate"

== system simpleVehicleModel_Trial2/Subsystem1/Track Segment Identifier ==
  1 if in first straight : Subsystem
  1 if in first turn : Subsystem
  1 if in last straight : Subsystem
  1 if in second turn : Subsystem
  1 if in transition phase : Subsystem
  Scope : Scope  NumInputPorts=5
  Out1 : Outport
  Out2 : Outport  Port=2
  Out3 : Outport  Port=3
  Out4 : Outport  Port=4
  Out5 : Outport  Port=5
  tag scope: S1=global, S2=global, S3=global, T1=global, T2=global
  wires:
  1 if in first turn/1(check turn 1) -> Scope/2, Out2/1, [T1]
  1 if in second turn/1(check turn 2) -> Scope/4, Out4/1, [T2]
  1 if in last straight/1(check last straight) -> Out5/1, [S3], Scope/5
  1 if in first straight/1(check straight 1) -> Scope/1, Out1/1, [S1]
  1 if in transition phase/1(check transition) -> Scope/3, Out3/1, [S2]

== system simpleVehicleModel_Trial2/Subsystem1/simple model ==
  steering_Angle : Inport
  Torque : Inport  Port=2
  Chassis : MATLAB Function  TreatAsAtomicUnit=on
  Delay : Delay  DelayLength=1  InitialCondition=[m*g*lr/(lf+lr)/2;m*g*lr/(lf+lr)/2;m*g*lf/(lf+lr)/2;m*g*lf/(lf+lr)/2]
  Delay1 : Delay  DelayLength=1  InitialCondition=[m*g*lr/(lf+lr)/2;m*g*lr/(lf+lr)/2;m*g*lf/(lf+lr)/2;m*g*lf/(lf+lr)/2]
  Delay2 : Delay  DelayLength=1
  Discrete-Time Integrator : DiscreteIntegrator  InitialCondition=60*5/18  InitialConditionSetting=State (most efficient)  SampleTime=-1  ICPrevOutput=DiscIntNeverNeededParam  ICPrevScaledInput=DiscIntNeverNeededParam
  Discrete-Time Integrator1 : DiscreteIntegrator  InitialConditionSetting=State (most efficient)  SampleTime=-1  ICPrevOutput=DiscIntNeverNeededParam  ICPrevScaledInput=DiscIntNeverNeededParam
  Discrete-Time Integrator2 : DiscreteIntegrator  InitialConditionSetting=State (most efficient)  SampleTime=-1  ICPrevOutput=DiscIntNeverNeededParam  ICPrevScaledInput=DiscIntNeverNeededParam
  Rate Limiter : RateLimiter  RisingSlewLimit=500*pi/180/12  FallingSlewLimit=-500*pi/180/12  SampleTimeMode=inherited
  Wheels : Subsystem  Priority=0
  Fz : Outport
  wires:
  [vx] -> Chassis/4(vx)
  Discrete-Time Integrator2/1 -> [yaw_Rate]
  [Fy] -> Chassis/2(Fy)
  [vy] -> Wheels/3(vy)
  [Torque] -> Wheels/1(Torque)
  [yaw_Rate] -> Wheels/4(yaw_Rate)
  [vx] -> Wheels/2(vx)
  [Fz] -> Wheels/6(Fz)
  [steering_Angle] -> Chassis/3(steeringAngle)
  [steering_Angle] -> Wheels/5(steering_Angle)
  steering_Angle/1 -> Rate Limiter/1
  Torque/1 -> [Torque]
  Chassis/5(yaw_Acc) -> Discrete-Time Integrator2/1
  Wheels/1(Fx) -> Delay/1  "Fx"
  Wheels/2(Fy) -> Delay1/1  "Fy"
  Chassis/6(Fz) -> Fz/1, [Fz]
  Delay/1 -> [Fx]
  Delay1/1 -> [Fy]
  Chassis/1(vx_dot) -> Discrete-Time Integrator/1
  Chassis/4(ay) -> [ay]
  Chassis/3(ax) -> [ax]
  Chassis/2(vy_dot) -> Discrete-Time Integrator1/1
  [vy] -> Chassis/5(vy)
  [yaw_Rate] -> Chassis/6(yaw_Rate)
  [Fx] -> Chassis/1(Fx)
  Discrete-Time Integrator1/1 -> [vy]
  Discrete-Time Integrator/1 -> [vx]
  Rate Limiter/1 -> Delay2/1
  Delay2/1 -> [steering_Angle]

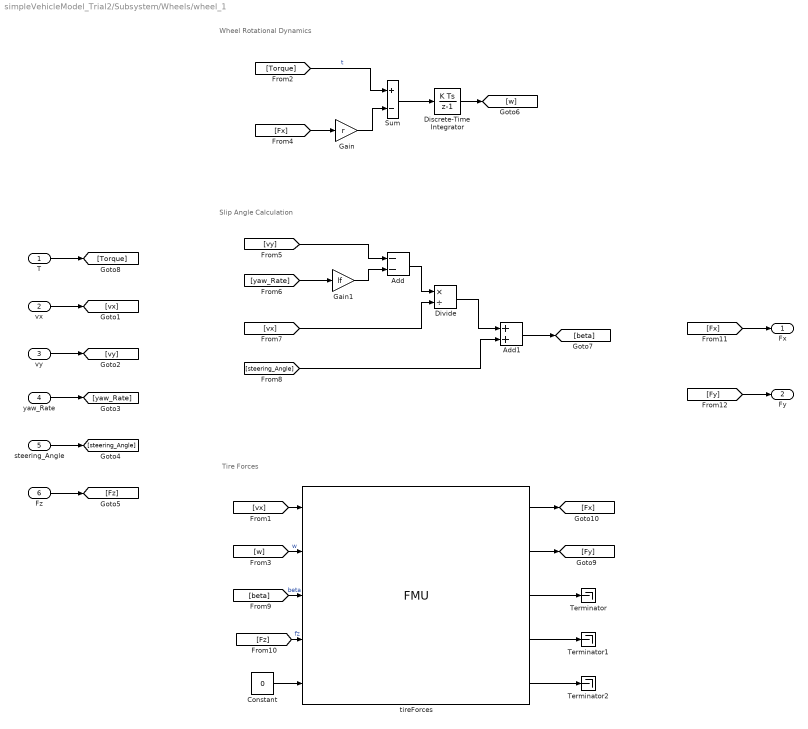
== system simpleVehicleModel_Trial2/Subsystem/Wheels/wheel_1 ==
  note: Tire Forces
  note: Wheel Rotational Dynamics
  note: Slip Angle Calculation
  T : Inport
  vx : Inport  Port=2
  vy : Inport  Port=3
  yaw_Rate : Inport  Port=4
  steering_Angle : Inport  Port=5
  Fz : Inport  Port=6
  Add : Sum  Inputs=--
  Add1 : Sum
  Constant : Constant  Value=0
  Discrete-Time Integrator : DiscreteIntegrator  InitialConditionSetting=State (most efficient)  SampleTime=-1  ICPrevOutput=DiscIntNeverNeededParam  ICPrevScaledInput=DiscIntNeverNeededParam
  Divide : Product  Inputs=*/
  Gain : Gain  Gain=r
  Gain1 : Gain  Gain=lf
  Sum : Sum  Inputs=+-
  Terminator : Terminator
  Terminator1 : Terminator
  Terminator2 : Terminator
  tireForces : FMU  FMUName=MED2018_TireModel.fmu  FMUMode=CoSimulation  FMUSampleTime=-1  mask(TyreFMUContainer [Co-Simulation, v2.0]){}
  Fx : Outport
  Fy : Outport  Port=2
  wires:
  Discrete-Time Integrator/1 -> [w]
  tireForces/5 -> Terminator2/1
  tireForces/2 -> [Fy]
  tireForces/4 -> Terminator1/1
  tireForces/3 -> Terminator/1
  Sum/1 -> Discrete-Time Integrator/1
  [Torque] -> Sum/1  "t"
  Gain/1 -> Sum/2
  [Fx] -> Gain/1
  Constant/1 -> tireForces/5
  Gain1/1 -> Add/2
  Add/1 -> Divide/1
  [w] -> tireForces/2  "w"
  vx/1 -> [vx]
  vy/1 -> [vy]
  steering_Angle/1 -> [steering_Angle]
  yaw_Rate/1 -> [yaw_Rate]
  Fz/1 -> [Fz]
  [vx] -> tireForces/1
  [vy] -> Add/1
  [yaw_Rate] -> Gain1/1
  [vx] -> Divide/2
  Divide/1 -> Add1/1
  [steering_Angle] -> Add1/2
  Add1/1 -> [beta]
  [beta] -> tireForces/3  "beta"
  [Fz] -> tireForces/4  "fz"
  T/1 -> [Torque]
  tireForces/1 -> [Fx]
  [Fx] -> Fx/1
  [Fy] -> Fy/1

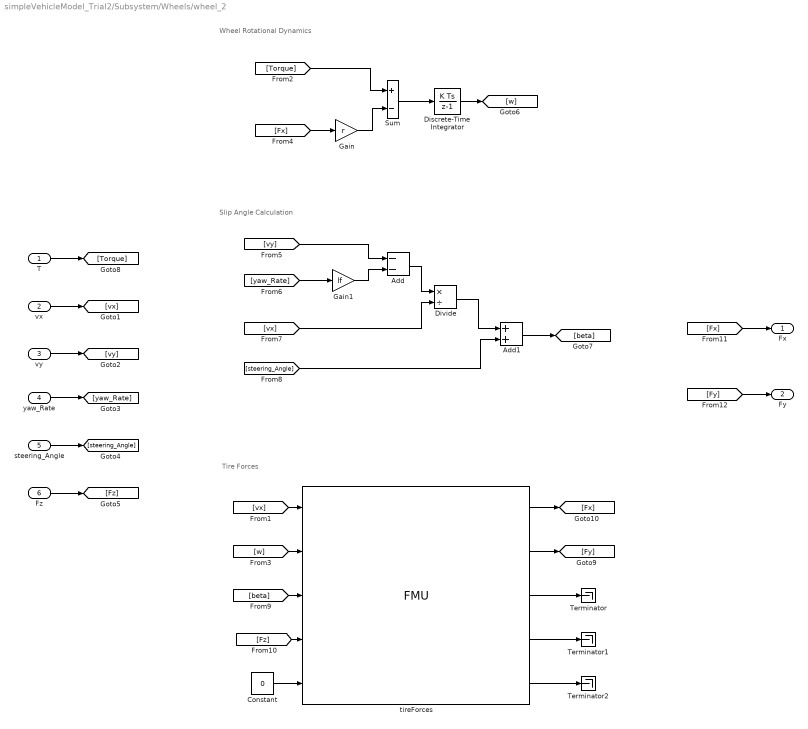
== system simpleVehicleModel_Trial2/Subsystem/Wheels/wheel_2 ==
  note: Tire Forces
  note: Wheel Rotational Dynamics
  note: Slip Angle Calculation
  T : Inport
  vx : Inport  Port=2
  vy : Inport  Port=3
  yaw_Rate : Inport  Port=4
  steering_Angle : Inport  Port=5
  Fz : Inport  Port=6
  Add : Sum  Inputs=--
  Add1 : Sum
  Constant : Constant  Value=0
  Discrete-Time Integrator : DiscreteIntegrator  InitialConditionSetting=State (most efficient)  SampleTime=-1  ICPrevOutput=DiscIntNeverNeededParam  ICPrevScaledInput=DiscIntNeverNeededParam
  Divide : Product  Inputs=*/
  Gain : Gain  Gain=r
  Gain1 : Gain  Gain=lf
  Sum : Sum  Inputs=+-
  Terminator : Terminator
  Terminator1 : Terminator
  Terminator2 : Terminator
  tireForces : FMU  FMUName=MED2018_TireModel.fmu  FMUMode=CoSimulation  FMUSampleTime=-1  mask(TyreFMUContainer [Co-Simulation, v2.0]){}
  Fx : Outport
  Fy : Outport  Port=2
  wires:
  Discrete-Time Integrator/1 -> [w]
  tireForces/5 -> Terminator2/1
  tireForces/2 -> [Fy]
  tireForces/4 -> Terminator1/1
  tireForces/3 -> Terminator/1
  Sum/1 -> Discrete-Time Integrator/1
  [Torque] -> Sum/1
  Gain/1 -> Sum/2
  [Fx] -> Gain/1
  Constant/1 -> tireForces/5
  Gain1/1 -> Add/2
  Add/1 -> Divide/1
  [w] -> tireForces/2
  vx/1 -> [vx]
  vy/1 -> [vy]
  steering_Angle/1 -> [steering_Angle]
  yaw_Rate/1 -> [yaw_Rate]
  Fz/1 -> [Fz]
  [vx] -> tireForces/1
  [vy] -> Add/1
  [yaw_Rate] -> Gain1/1
  [vx] -> Divide/2
  Divide/1 -> Add1/1
  [steering_Angle] -> Add1/2
  Add1/1 -> [beta]
  [beta] -> tireForces/3
  [Fz] -> tireForces/4
  T/1 -> [Torque]
  tireForces/1 -> [Fx]
  [Fx] -> Fx/1
  [Fy] -> Fy/1

== system simpleVehicleModel_Trial2/Subsystem/Wheels/wheel_3 ==
  note: Tire Forces
  note: Wheel Rotational Dynamics
  note: Slip Angle Calculation
  T : Inport
  vx : Inport  Port=2
  vy : Inport  Port=3
  yaw_Rate : Inport  Port=4
  Fz : Inport  Port=5
  Add : Sum  Inputs=-+
  Constant : Constant  Value=0
  Discrete-Time Integrator : DiscreteIntegrator  InitialConditionSetting=State (most efficient)  SampleTime=-1  ICPrevOutput=DiscIntNeverNeededParam  ICPrevScaledInput=DiscIntNeverNeededParam
  Divide : Product  Inputs=*/
  Gain : Gain  Gain=r
  Gain1 : Gain  Gain=lr
  Sum : Sum  Inputs=+-
  Terminator : Terminator
  Terminator1 : Terminator
  Terminator2 : Terminator
  tireForces : FMU  FMUName=MED2018_TireModel.fmu  FMUMode=CoSimulation  FMUSampleTime=-1  mask(TyreFMUContainer [Co-Simulation, v2.0]){}
  Fx : Outport
  Fy : Outport  Port=2
  wires:
  Discrete-Time Integrator/1 -> [w]
  tireForces/5 -> Terminator2/1
  tireForces/2 -> [Fy]
  tireForces/4 -> Terminator1/1
  tireForces/3 -> Terminator/1
  Sum/1 -> Discrete-Time Integrator/1
  [Torque] -> Sum/1
  Gain/1 -> Sum/2
  [Fx] -> Gain/1
  Constant/1 -> tireForces/5
  Gain1/1 -> Add/2
  Add/1 -> Divide/1
  [w] -> tireForces/2
  vx/1 -> [vx]
  vy/1 -> [vy]
  yaw_Rate/1 -> [yaw_Rate]
  Fz/1 -> [Fz]
  [vx] -> tireForces/1
  [vy] -> Add/1
  [yaw_Rate] -> Gain1/1
  [vx] -> Divide/2
  [beta] -> tireForces/3
  [Fz] -> tireForces/4
  T/1 -> [Torque]
  tireForces/1 -> [Fx]
  [Fx] -> Fx/1
  [Fy] -> Fy/1
  Divide/1 -> [beta]

== system simpleVehicleModel_Trial2/Subsystem/Wheels/wheel_4 ==
  note: Tire Forces
  note: Wheel Rotational Dynamics
  note: Slip Angle Calculation
  T : Inport
  vx : Inport  Port=2
  vy : Inport  Port=3
  yaw_Rate : Inport  Port=4
  Fz : Inport  Port=5
  Add : Sum  Inputs=-+
  Constant : Constant  Value=0
  Discrete-Time Integrator : DiscreteIntegrator  InitialConditionSetting=State (most efficient)  SampleTime=-1  ICPrevOutput=DiscIntNeverNeededParam  ICPrevScaledInput=DiscIntNeverNeededParam
  Divide : Product  Inputs=*/
  Gain : Gain  Gain=r
  Gain1 : Gain  Gain=lr
  Sum : Sum  Inputs=+-
  Terminator : Terminator
  Terminator1 : Terminator
  Terminator2 : Terminator
  tireForces : FMU  FMUName=MED2018_TireModel.fmu  FMUDebugLogging=on  FMUMode=CoSimulation  FMUSampleTime=-1  mask(TyreFMUContainer [Co-Simulation, v2.0]){}
  Fx : Outport
  Fy : Outport  Port=2
  wires:
  Discrete-Time Integrator/1 -> [w]
  tireForces/5 -> Terminator2/1
  tireForces/2 -> [Fy]
  tireForces/4 -> Terminator1/1
  tireForces/3 -> Terminator/1
  Sum/1 -> Discrete-Time Integrator/1
  [Torque] -> Sum/1
  Gain/1 -> Sum/2
  [Fx] -> Gain/1
  Constant/1 -> tireForces/5
  [w] -> tireForces/2
  vx/1 -> [vx]
  vy/1 -> [vy]
  yaw_Rate/1 -> [yaw_Rate]
  Fz/1 -> [Fz]
  [vx] -> tireForces/1
  [beta] -> tireForces/3
  [Fz] -> tireForces/4
  T/1 -> [Torque]
  tireForces/1 -> [Fx]
  [Fx] -> Fx/1
  [Fy] -> Fy/1
  [vy] -> Add/1
  [vx] -> Divide/2
  [yaw_Rate] -> Gain1/1
  Add/1 -> Divide/1
  Gain1/1 -> Add/2
  Divide/1 -> [beta]

== system simpleVehicleModel_Trial2/Subsystem1/S1/Wheel Traction control ==
  cmd_Tx : Inport
  Fmargin : Inport  Port=2
  Abs{,1..3} (4 alike) : Abs
  Demux : Demux
  Min{,1..3} (4 alike) : MinMax  Inputs=2
  Product{,1..3} (4 alike) : Product
  Sign{,1..3} (4 alike) : Signum
  cmd_Tx_FL : Outport
  cmd_Tx_FR : Outport  Port=2
  cmd_Tx_RL : Outport  Port=3
  cmd_Tx_RR : Outport  Port=4
  wires:
  Abs/1 -> Min/1
  cmd_Tx/1 -> [cmd_Tx]
  Min/1 -> Product/2
  Sign/1 -> Product/1
  Product/1 -> cmd_Tx_FL/1
  [cmd_Tx] -> Abs/1, Sign/1
  Fmargin/1 -> Demux/1
  Demux/1 -> [Fmargin_1]
  Demux/2 -> [Fmargin_2]
  Demux/3 -> [Fmargin_3]
  Demux/4 -> [Fmargin_4]
  [Fmargin_1] -> Min/2
  Min1/1 -> Product1/2
  Abs1/1 -> Min1/1
  [cmd_Tx] -> Abs1/1, Sign1/1
  Product1/1 -> cmd_Tx_RL/1
  Sign1/1 -> Product1/1
  [Fmargin_3] -> Min1/2
  [Fmargin_2] -> Min2/2
  Sign2/1 -> Product2/1
  Product2/1 -> cmd_Tx_FR/1
  [cmd_Tx] -> Sign2/1, Abs2/1
  Abs2/1 -> Min2/1
  Min2/1 -> Product2/2
  Min3/1 -> Product3/2
  Abs3/1 -> Min3/1
  [cmd_Tx] -> Abs3/1, Sign3/1
  Product3/1 -> cmd_Tx_RR/1
  Sign3/1 -> Product3/1
  [Fmargin_4] -> Min3/2

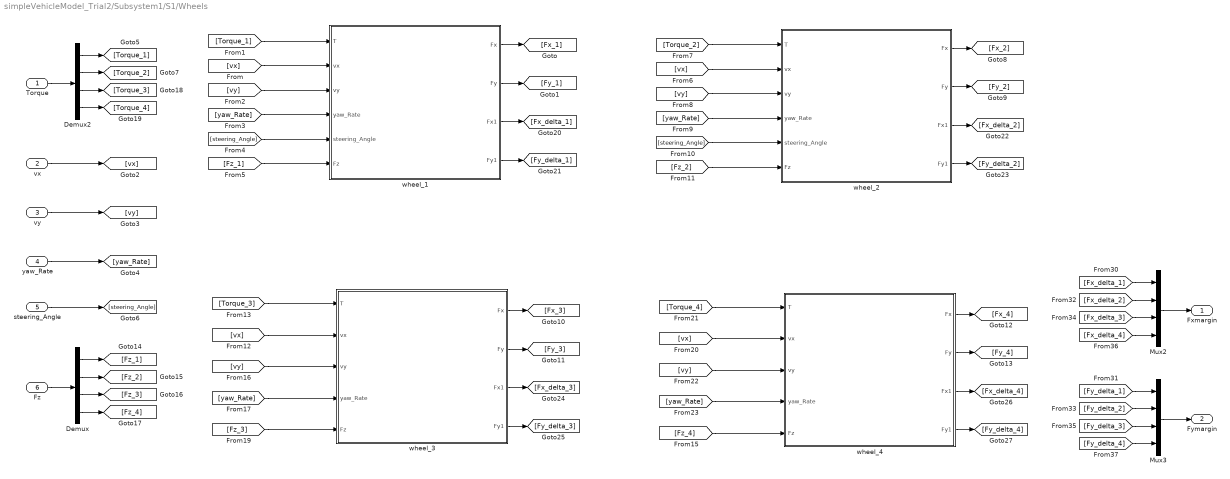
== system simpleVehicleModel_Trial2/Subsystem1/S1/Wheels ==
  Torque : Inport
  vx : Inport  Port=2
  vy : Inport  Port=3
  yaw_Rate : Inport  Port=4
  steering_Angle : Inport  Port=5
  Fz : Inport  Port=6
  Demux : Demux
  Demux2 : Demux
  Mux2 : Mux
  Mux3 : Mux
  wheel_1 : Subsystem
  wheel_2 : Subsystem
  wheel_3 : Subsystem
  wheel_4 : Subsystem
  Fxmargin : Outport
  Fymargin : Outport  Port=2
  wires:
  vx/1 -> [vx]
  vy/1 -> [vy]
  yaw_Rate/1 -> [yaw_Rate]
  [vx] -> wheel_1/2(vx)
  wheel_1/1(Fx) -> [Fx_1]
  wheel_1/2(Fy) -> [Fy_1]
  [steering_Angle] -> wheel_1/5(steering_Angle)
  [yaw_Rate] -> wheel_1/4(yaw_Rate)
  [vy] -> wheel_1/3(vy)
  [Torque_1] -> wheel_1/1(T)
  steering_Angle/1 -> [steering_Angle]
  wheel_2/1(Fx) -> [Fx_2]
  wheel_2/2(Fy) -> [Fy_2]
  [yaw_Rate] -> wheel_2/4(yaw_Rate)
  [vy] -> wheel_2/3(vy)
  [steering_Angle] -> wheel_2/5(steering_Angle)
  [vx] -> wheel_2/2(vx)
  wheel_3/1(Fx) -> [Fx_3]
  [yaw_Rate] -> wheel_3/4(yaw_Rate)
  [vy] -> wheel_4/3(vy)
  [yaw_Rate] -> wheel_4/4(yaw_Rate)
  [vx] -> wheel_4/2(vx)
  wheel_4/2(Fy) -> [Fy_4]
  wheel_3/2(Fy) -> [Fy_3]
  wheel_4/1(Fx) -> [Fx_4]
  [vy] -> wheel_3/3(vy)
  [vx] -> wheel_3/2(vx)
  Demux/1 -> [Fz_1]
  Demux/2 -> [Fz_2]
  Demux/3 -> [Fz_3]
  Demux/4 -> [Fz_4]
  [Fz_1] -> wheel_1/6(Fz)
  [Fz_3] -> wheel_3/5(Fz)
  [Fz_4] -> wheel_4/5(Fz)
  [Fz_2] -> wheel_2/6(Fz)
  Fz/1 -> Demux/1
  [Torque_3] -> wheel_3/1(T)
  [Torque_2] -> wheel_2/1(T)
  [Torque_4] -> wheel_4/1(T)
  Demux2/4 -> [Torque_4]
  Demux2/3 -> [Torque_3]
  Demux2/1 -> [Torque_1]
  Torque/1 -> Demux2/1
  Demux2/2 -> [Torque_2]
  wheel_4/4(Fy1) -> [Fy_delta_4]
  wheel_4/3(Fx1) -> [Fx_delta_4]
  wheel_3/3(Fx1) -> [Fx_delta_3]
  wheel_1/4(Fy1) -> [Fy_delta_1]
  wheel_2/3(Fx1) -> [Fx_delta_2]
  wheel_2/4(Fy1) -> [Fy_delta_2]
  wheel_1/3(Fx1) -> [Fx_delta_1]
  wheel_3/4(Fy1) -> [Fy_delta_3]
  [Fx_delta_4] -> Mux2/4
  [Fy_delta_1] -> Mux3/1
  [Fy_delta_4] -> Mux3/4
  [Fy_delta_2] -> Mux3/2
  [Fx_delta_3] -> Mux2/3
  Mux3/1 -> Fymargin/1
  [Fx_delta_2] -> Mux2/2
  Mux2/1 -> Fxmargin/1
  [Fx_delta_1] -> Mux2/1
  [Fy_delta_3] -> Mux3/3

== system simpleVehicleModel_Trial2/Subsystem1/Track Segment Identifier/1 if in first straight ==
  Check Dynamic Range : simulink/Model Verification/Check  Dynamic Range  Description=min < u < max  enabled=off  stopWhenAssertionFail=off  export=on  icon=graphic
      settings: SourceProductName=Simulink  SourceProductBaseCode=SL
  Check Dynamic Range1 : simulink/Model Verification/Check  Dynamic Range  Description=min < u < max  enabled=off  stopWhenAssertionFail=off  export=on  icon=graphic
      settings: SourceProductName=Simulink  SourceProductBaseCode=SL
  Constant : Constant  Value=50
  Constant1 : Constant  Value=0
  Constant2 : Constant  Value=6
  Constant3 : Constant  Value=-6
  Logical Operator : Logic  AllPortsSameDT=off  OutDataTypeStr=boolean
  check straight 1 : Outport
  wires:
  [Y] -> Check Dynamic Range1/3
  Check Dynamic Range1/1 -> Logical Operator/2
  Constant1/1 -> Check Dynamic Range/2
  [X] -> Check Dynamic Range/3
  Check Dynamic Range/1 -> Logical Operator/1
  Constant3/1 -> Check Dynamic Range1/2
  Constant2/1 -> Check Dynamic Range1/1
  Logical Operator/1 -> check straight 1/1
  Constant/1 -> Check Dynamic Range/1

== system simpleVehicleModel_Trial2/Subsystem1/Track Segment Identifier/1 if in first turn ==
  Check Dynamic Range : simulink/Model Verification/Check  Dynamic Range  Description=min < u < max  enabled=off  stopWhenAssertionFail=off  export=on  icon=graphic
      settings: SourceProductName=Simulink  SourceProductBaseCode=SL
  Check Dynamic Range1 : simulink/Model Verification/Check  Dynamic Range  Description=min < u < max  enabled=off  stopWhenAssertionFail=off  export=on  icon=graphic
      settings: SourceProductName=Simulink  SourceProductBaseCode=SL
  Constant : Constant  Value=106
  Constant1 : Constant  Value=50
  Constant2 : Constant  Value=106
  Constant3 : Constant  Value=-6
  Logical Operator : Logic  AllPortsSameDT=off  OutDataTypeStr=boolean
  check turn 1 : Outport
  wires:
  Constant/1 -> Check Dynamic Range/1
  Logical Operator/1 -> check turn 1/1
  Constant2/1 -> Check Dynamic Range1/1
  Constant3/1 -> Check Dynamic Range1/2
  Check Dynamic Range/1 -> Logical Operator/1
  [X] -> Check Dynamic Range/3
  Constant1/1 -> Check Dynamic Range/2
  Check Dynamic Range1/1 -> Logical Operator/2
  [Y] -> Check Dynamic Range1/3

== system simpleVehicleModel_Trial2/Subsystem1/Track Segment Identifier/1 if in last straight ==
  Check Dynamic Range : simulink/Model Verification/Check  Dynamic Range  Description=min < u < max  enabled=off  stopWhenAssertionFail=off  export=on  icon=graphic
      settings: SourceProductName=Simulink  SourceProductBaseCode=SL
  Check Dynamic Range1 : simulink/Model Verification/Check  Dynamic Range  Description=min < u < max  enabled=off  stopWhenAssertionFail=off  export=on  icon=graphic
      settings: SourceProductName=Simulink  SourceProductBaseCode=SL
  Constant : Constant  Value=120
  Constant1 : Constant  Value=50
  Constant2 : Constant  Value=176
  Constant3 : Constant  Value=164
  Logical Operator : Logic  AllPortsSameDT=off  OutDataTypeStr=boolean
  check last straight : Outport
  wires:
  [Y] -> Check Dynamic Range1/3
  Check Dynamic Range1/1 -> Logical Operator/2
  Constant1/1 -> Check Dynamic Range/2
  [X] -> Check Dynamic Range/3
  Check Dynamic Range/1 -> Logical Operator/1
  Constant3/1 -> Check Dynamic Range1/2
  Constant2/1 -> Check Dynamic Range1/1
  Logical Operator/1 -> check last straight/1
  Constant/1 -> Check Dynamic Range/1

== system simpleVehicleModel_Trial2/Subsystem1/Track Segment Identifier/1 if in second turn ==
  Check Dynamic Range : simulink/Model Verification/Check  Dynamic Range  Description=min < u < max  enabled=off  stopWhenAssertionFail=off  export=on  icon=graphic
      settings: SourceProductName=Simulink  SourceProductBaseCode=SL
  Check Dynamic Range1 : simulink/Model Verification/Check  Dynamic Range  Description=min < u < max  enabled=off  stopWhenAssertionFail=off  export=on  icon=graphic
      settings: SourceProductName=Simulink  SourceProductBaseCode=SL
  Constant : Constant  Value=50
  Constant1 : Constant  Value=9
  Constant2 : Constant  Value=182
  Constant3 : Constant  Value=100
  Logical Operator : Logic  AllPortsSameDT=off  OutDataTypeStr=boolean
  check turn 2 : Outport
  wires:
  Constant/1 -> Check Dynamic Range/1
  Logical Operator/1 -> check turn 2/1
  Constant2/1 -> Check Dynamic Range1/1
  Constant3/1 -> Check Dynamic Range1/2
  Check Dynamic Range/1 -> Logical Operator/1
  [X] -> Check Dynamic Range/3
  Constant1/1 -> Check Dynamic Range/2
  Check Dynamic Range1/1 -> Logical Operator/2
  [Y] -> Check Dynamic Range1/3
